simulink model "Event6"  (R2020b)
settings: Solver=FixedStepDiscrete  StartTime=0.0  StopTime=0.1  FixedStep=0.1  RelTol=1e-3  EnableMultiTasking=on
settings Model: Creator=BEAR  LastModifiedBy=apple
settings SolverCC: AutoInsertRateTranBlk=on
settings DataIOCC: LimitDataPoints=on  ReturnWorkspaceOutputs=off
settings OptimizationCC: LifeSpan=inf
settings DebuggingCC: AllowSymbolicDim=off  SFUnexpectedBacktrackingDiag=warning  SFNoUnconditionalDefaultTransitionDiag=warning  SFExecutionAtInitializationDiag=none  ArithmeticOperatorsInVariantConditions=warning
settings SFSimCC: SimUseLocalCustomCode=off  CustomCodeUndefinedFunction=UseInterfaceOnly
settings RTWCC: RTWUseLocalCustomCode=off
settings CodeAppCC: StateflowObjectComments=on
settings GRTTargetCC: TargetLangStandard=C89/C90 (ANSI)
settings ConfigComp: CovMetricSettings=dw  CovSaveCumulativeToWorkspaceVar=on  CovSaveSingleToWorkspaceVar=on  CovExternalEMLEnable=off  CovSFcnEnable=off

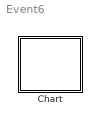
== system Event6 ==
  Chart : Stateflow chart  TreatAsAtomicUnit=on

== stateflow chart Event6/Chart ==
  state A [parallel]
    settings: executionOrder=1
    state A1
    state A2
    (default) -> A1
    A1 -> A2 : /{E}
  state B [parallel]
    settings: executionOrder=2
    state B1
    state B2
      en: fprintf("en_A2")
    (default) -> B1 : {x=6;}
    B1 -> B2 : E[x>0]{x=x-1;fprintf("a");E}
  data: x local int32
  events: E local FUNCTION_CALL_EVENT
